simulink model "controller_ballcatcher_inv_kin_mind_timestamp"  (R2018b)
settings: Solver=FixedStepDiscrete  StartTime=0.0  StopTime=10.0  FixedStep=timing.T_optiTask  RelTol=1e-3
InitFcn:
  | iiwa_joint_trajectoryfollowingcontrol_rigid_parameters;
values from neighbouring files (symbols this model uses):
  estimator_init_struct = struct()    [init_estimator_struct.m]
  filter_tau_p_slow_T_1 = filter_tau_slow_T_1    [parameters.m]
  filter_tau_slow_T_1 = 1./(2*pi*[200;200;200;200;200;200;200])    [parameters.m]
  filter_theta_p_slow_T_1 = filter_tau_slow_T_1    [parameters.m]
  filter_theta_slow_T_1 = filter_tau_slow_T_1    [parameters.m]
  height_of_catch = 0.9    [init_estimator_struct.m]
  optitrack_data = struct()    [init_parabola.m]
  param_robot = struct()    [parameters.m]
  positions = struct()    [init_common_positions.m]
  sensor_torque_offset = [0.53;-0.095;-0.189;0.07;-0.058;0.0025;-0.12]    [parameters.m]
  timing = struct()    [parameters.m]
undefined symbols (not defined in the file or in its folder): param_controller
settings Model: TCT_ExtModeMexArgs=[128 131 86 77 1 1],16842832  SimulationMode=external  Creator=cha  LastModifiedBy=student
settings SolverCC: AutoInsertRateTranBlk=on
settings DataIOCC: LoggingToFile=on  LoggingFileName=benniii.mat
settings OptimizationCC: UseFloatMulNetSlope=on  PassReuseOutputArgsThreshold=0  LocalBlockOutputs=off  EfficientFloat2IntCast=on  OptimizeBlockOrder=speed  DifferentSizesBufferReuse=on
settings DebuggingCC: ParameterTunabilityLossMsg=error
settings HardwareCC: ProdLongLongMode=on
settings ModelReferenceCC: EnableParallelModelReferenceBuilds=on  ModelReferenceNumInstancesAllowed=Single
settings SFSimCC: SimUseLocalCustomCode=off  MATLABDynamicMemAlloc=off
settings RTWCC: SystemTargetFile=TwinCAT.tlc  GenCodeOnly=on  MakeCommand=make_tct  TemplateMakefile=tct_msbuild.tmf  Description=TwinCAT Target  GenerateReport=on  RTWUseLocalCustomCode=off  TargetLang=C++
settings RTWCC: CustomHeaderCode=|
  | #define fflush(stdout)
  | #define printf(...) m_spSrv->TcReportLog(ADSLOG_MSGTYPE_LOG,__VA_ARGS__)
settings CodeAppCC: ForceParamTrailComments=on  MaxIdLength=47  OperatorAnnotations=on  StateflowObjectComments=on  MATLABSourceComments=on
settings STFCustomTargetCC: TargetLangStandard=C++03 (ISO)  CompOptLevelCompliant=on  MATLABClassNameForMDSCustomization=Simulink.SoftwareTarget.TargetSpecificTriggerConfigurationBase  GRTInterface=on  SystemTargetFile=TwinCAT.tlc

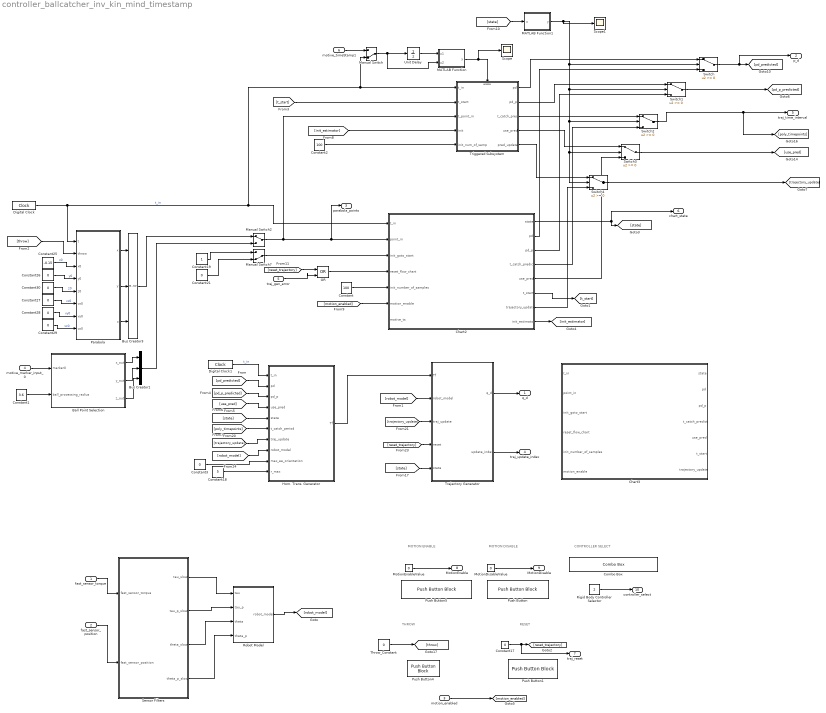
== system controller_ballcatcher_inv_kin_mind_timestamp ==
  note: THROW
  note: RESET
  note: MOTION ENABLE
  note: MOTION DISABLE
  note: CONTROLLER SELECT
  fast_sensor_torque : Inport
  fast_sensor_position : Inport  Port=2
  motion_enabled : Inport  Port=3
  motive_marker_input_0 : Inport  Port=4  OutDataTypeStr=Bus: Marker
  traj_gen_error : Inport  Port=5  OutDataTypeStr=boolean
  motive_timeStamp1 : Inport  Port=6
  Ball Point Selection : MATLAB Function  TreatAsAtomicUnit=on
  Bus Creator1 : BusCreator  Inputs=3
  Bus Creator3 : BusCreator  Inputs=3
  Chart2 : Stateflow chart  TreatAsAtomicUnit=on
  Chart3 : Subsystem
      mask help: Simulink:masks:GenSFuncDesc_MD
      mask Help: eval('feval(''rtwprivate'',''rtwhelpview'',''rtw_sfcn_block'')');
  Combo Box : ComboBox  WebBlockId=3098  SelectedLabel=2: Joint-based E/A Linearization
      settings: Values={{'1: Gravity Compensation q-based', '2: Joint-based E/A Linearization'}, [1 2]}
  Constant : Constant  Value=100
  Constant1 : Constant  Value=3.6
  Constant{3,17,21,26..30} (8 alike) : Constant  Value=0
  Constant18 : Constant  Value=5
  Constant19 : Constant
  Constant2 : Constant  Value=100
  Constant25 : Constant  Value=-0.15
  Digital Clock : DigitalClock  SampleTime=timing.T_optitrack
  Digital Clock1 : DigitalClock  SampleTime=timing.T_optiTask
  Hom. Trans. Generator : MATLAB Function  TreatAsAtomicUnit=on
  MATLAB Function : MATLAB Function  TreatAsAtomicUnit=on
  MATLAB Function1 : MATLAB Function  TreatAsAtomicUnit=on
  Manual Switch : ManualSwitch  CurrentSetting=0
  Manual Switch2 : ManualSwitch
  Manual Switch7 : ManualSwitch  CurrentSetting=0
  MotionDisableValue : Constant  Value=0
  MotionEnableValue : Constant  Value=0
  OR : Logic  Operator=OR  IconShape=distinctive  AllPortsSameDT=off  OutDataTypeStr=boolean
  Parabola : MATLAB Function  TreatAsAtomicUnit=on
  Push Button : PushButtonBlock  WebBlockId=3092  ButtonText=Motion disable
  Push Button1 : PushButtonBlock  WebBlockId=1355  ButtonText=Reset Trajectory
  Push Button4 : PushButtonBlock  WebBlockId=2019  ButtonText=Throw
  Push Button5 : PushButtonBlock  WebBlockId=3093  ButtonText=Motion enable
  Rigid Body Controller Selector : Constant  Value=2  OutDataTypeStr=uint32
  Robot Model : MATLAB Function  TreatAsAtomicUnit=on
  Scope : Scope
  Scope1 : Scope
  Sensor Filters : Subsystem
  Switch{,2..4} (4 alike) : Switch
  Switch1 : Switch  InputSameDT=on
  Throw_Constant : Constant  Value=0
  Trajectory Generator : MATLAB Function  TreatAsAtomicUnit=on
  Triggered Subsystem : Subsystem  TreatAsAtomicUnit=on
  Unit Delay : UnitDelay  SampleTime=-1
  q_d : Outport  PortDimensions=7  VectorParamsAs1DForOutWhenUnconnected=on
  p_d : Outport  Port=2  VectorParamsAs1DForOutWhenUnconnected=on
  parabola_points : Outport  Port=3  VectorParamsAs1DForOutWhenUnconnected=on
  traj_update_index : Outport  Port=4
  traj_time_interval : Outport  Port=5
  chart_state : Outport  Port=6
  traj_reset : Outport  Port=7
  MotionEnable : Outport  Port=8
  MotionDisable : Outport  Port=9
  controller_select : Outport  Port=10
  wires:
  motion_enabled/1 -> [motion_enabled]
  fast_sensor_torque/1 -> Sensor Filters/1(fast_sensor_torque)
  fast_sensor_position/1 -> Sensor Filters/2(fast_sensor_position)
  Sensor Filters/1(tau_slow) -> Robot Model/1(tau)
  Sensor Filters/2(tau_p_slow) -> Robot Model/2(tau_p)
  Sensor Filters/3(theta_slow) -> Robot Model/3(theta)
  Sensor Filters/4(theta_p_slow) -> Robot Model/4(theta_p)
  Robot Model/1(robot_model) -> [robot_model]
  [use_pred] -> Hom. Trans. Generator/4(use_pred)
  [pd_p_predicted] -> Hom. Trans. Generator/3(pd_p)
  [state] -> Hom. Trans. Generator/5(state)
  [pd_predicted] -> Hom. Trans. Generator/2(pd)
  Constant21/1 -> Manual Switch7/2
  Constant19/1 -> Manual Switch7/1
  motive_marker_input_0/1 -> Ball Point Selection/1(marker0)
  Hom. Trans. Generator/1(Tf) -> Trajectory Generator/1(Tf)
  Trajectory Generator/1(q_d) -> q_d/1
  Manual Switch7/1 -> Chart2/3(init_goto_start)
  Chart2/1(state) -> [state], chart_state/1
  Chart2/6(t_start) -> [t_start]
  Digital Clock/1 -> Manual Switch/2, Triggered Subsystem/1(t_in), Chart2/1(t_in), Parabola/1(t)  "t_in"
  Ball Point Selection/1(x_out) -> Bus Creator1/1
  Ball Point Selection/2(y_out) -> Bus Creator1/2
  Ball Point Selection/3(z_out) -> Bus Creator1/3
  [throw] -> Parabola/2(throw)
  Throw_Constant/1 -> [throw]
  Parabola/3(z) -> Bus Creator3/3
  Parabola/2(y) -> Bus Creator3/2
  Parabola/1(x) -> Bus Creator3/1
  Manual Switch2/1 -> Triggered Subsystem/3(t_point_in), Chart2/2(point_in), parabola_points/1
  Bus Creator3/1 -> Manual Switch2/1
  Bus Creator1/1 -> Manual Switch2/2
  Constant26/1 -> Parabola/4(y0)  "y0"
  Constant27/1 -> Parabola/6(vx0)  "vx0"
  Constant30/1 -> Parabola/5(z0)  "z0"
  Constant25/1 -> Parabola/3(x0)  "x0"
  Constant29/1 -> Parabola/8(vz0)  "vz0"
  Constant28/1 -> Parabola/7(vy0)  "vy0"
  [poly_timepoints] -> Hom. Trans. Generator/6(t_catch_period)
  [trajectory_update] -> Trajectory Generator/3(traj_update)
  [robot_model] -> Hom. Trans. Generator/8(robot_model)
  Constant/1 -> Chart2/5(init_number_of_samples)
  [trajectory_update] -> Hom. Trans. Generator/7(traj_update)
  Constant1/1 -> Ball Point Selection/2(ball_processing_radius)
  Constant3/1 -> Hom. Trans. Generator/9(max_ee_orientation)
  [reset_trajectory] -> Trajectory Generator/4(reset)
  [motion_enabled] -> Chart2/6(motion_enable)
  Constant18/1 -> Hom. Trans. Generator/10(r_max)
  [state] -> Trajectory Generator/5(state)
  Constant17/1 -> traj_reset/1, [reset_trajectory]
  OR/1 -> Chart2/4(reset_flow_chart)
  [reset_trajectory] -> OR/1
  traj_gen_error/1 -> OR/2
  Trajectory Generator/2(update_index) -> traj_update_index/1
  Digital Clock1/1 -> Hom. Trans. Generator/1(t_in)  "t_in"
  [robot_model] -> Trajectory Generator/2(robot_model)
  MotionDisableValue/1 -> MotionDisable/1
  MotionEnableValue/1 -> MotionEnable/1
  Rigid Body Controller Selector/1 -> controller_select/1
  [t_start] -> Triggered Subsystem/2(t_start)
  Chart2/8(init_estimator) -> [init_estimator]
  [init_estimator] -> Triggered Subsystem/4(init)
  Constant2/1 -> Triggered Subsystem/5(init_num_of_samp)
  Unit Delay/1 -> MATLAB Function/1(u1)
  Switch/1 -> p_d/1, [pd_predicted]
  Switch1/1 -> [pd_p_predicted]
  Switch2/1 -> [poly_timepoints], traj_time_interval/1
  Switch3/1 -> [use_pred]
  Triggered Subsystem/1(pd) -> Switch/1
  Triggered Subsystem/2(pd_p) -> Switch1/1
  Triggered Subsystem/4(use_pred) -> Switch3/1
  Triggered Subsystem/3(t_catch_pred) -> Switch2/1
  Triggered Subsystem/5(pred_update) -> Switch4/1
  Switch4/1 -> [trajectory_update]
  Chart2/2(pd) -> Switch/3
  Chart2/3(pd_p) -> Switch1/3
  Chart2/4(t_catch_predict) -> Switch2/3
  Chart2/5(use_pred) -> Switch3/3
  Chart2/7(trajectory_update) -> Switch4/3
  [state] -> MATLAB Function1/1(u)
  MATLAB Function1/1(y) -> Scope1/1, Switch4/2, Switch3/2, Switch2/2, Switch1/2, Switch/2
  MATLAB Function/1(y) -> Triggered Subsystem/Enable, Scope/1
  Manual Switch/1 -> Unit Delay/1, MATLAB Function/2(u2)
  motive_timeStamp1/1 -> Manual Switch/1

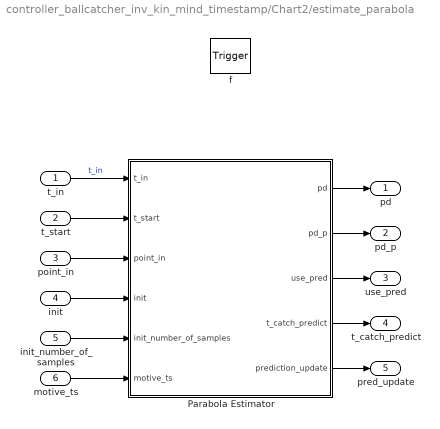
== system controller_ballcatcher_inv_kin_mind_timestamp/Chart2/estimate_parabola ==
  t_in : Inport  OutDataTypeStr=double  PortDimensions=1
  t_start : Inport  Port=2  OutDataTypeStr=double  PortDimensions=1
  point_in : Inport  Port=3  OutDataTypeStr=double  PortDimensions=3
  init : Inport  Port=4  OutDataTypeStr=double  PortDimensions=1
  init_number_of_samples : Inport  Port=5  OutDataTypeStr=double  PortDimensions=1
  motive_ts : Inport  Port=6  OutDataTypeStr=double  PortDimensions=1
  f : TriggerPort  TriggerType=function-call  VariantControl=(inherit)
      settings: CopyFcn=Stateflow.SLINSF.SimulinkMan.removeBlockPreDeleteFcn  PreDeleteFcn=Stateflow.SLINSF.SimulinkMan.unsafePredeleteFcn
  Parabola Estimator : MATLAB Function  TreatAsAtomicUnit=on
  pd : Outport  PortDimensions=3  VectorParamsAs1DForOutWhenUnconnected=on
  pd_p : Outport  Port=2  PortDimensions=3  VectorParamsAs1DForOutWhenUnconnected=on
  use_pred : Outport  Port=3  PortDimensions=1  VectorParamsAs1DForOutWhenUnconnected=on
  t_catch_predict : Outport  Port=4  PortDimensions=[1,2]  VectorParamsAs1DForOutWhenUnconnected=on
  pred_update : Outport  Port=5  VectorParamsAs1DForOutWhenUnconnected=on
  wires:
  init_number_of_samples/1 -> Parabola Estimator/5(init_number_of_samples)
  Parabola Estimator/5(prediction_update) -> pred_update/1
  init/1 -> Parabola Estimator/4(init)
  t_start/1 -> Parabola Estimator/2(t_start)
  point_in/1 -> Parabola Estimator/3(point_in)
  t_in/1 -> Parabola Estimator/1(t_in)  "t_in"
  Parabola Estimator/3(use_pred) -> use_pred/1
  Parabola Estimator/4(t_catch_predict) -> t_catch_predict/1
  Parabola Estimator/1(pd) -> pd/1
  Parabola Estimator/2(pd_p) -> pd_p/1
  motive_ts/1 -> Parabola Estimator/6(motive_ts)

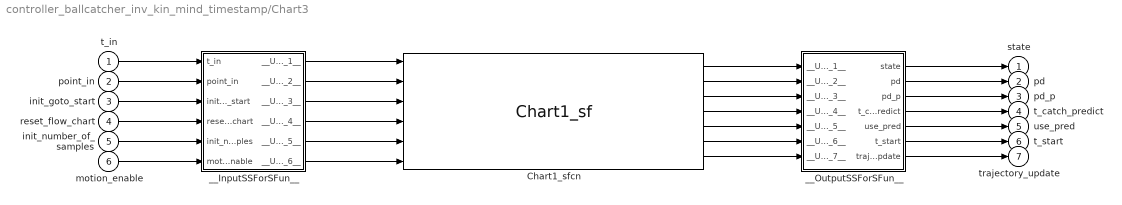
== system controller_ballcatcher_inv_kin_mind_timestamp/Chart3 ==
  t_in : Inport
  point_in : Inport  Port=2
  init_goto_start : Inport  Port=3
  reset_flow_chart : Inport  Port=4
  init_number_of_samples : Inport  Port=5
  motion_enable : Inport  Port=6
  Chart1_sfcn : S-Function  FunctionName=Chart1_sf  SFunctionModules=""  SFunctionDeploymentMode=off  EnableBusSupport=off  mask{rtw_sf_name=Chart1_sf, showVar=off}
      mask prompts: rtw_sf_name "Simulink:masks:GenSFuncName_MP"; showVar "Simulink:masks:GenSFuncShowModuleList_MP"
      mask help: Simulink:masks:GenSFuncDesc_MD
      mask init:
      | displist = '';
      | if ~strcmp(get_param(gcb, 'FunctionName'), rtw_sf_name);
      |   set_param(gcb, 'FunctionName', rtw_sf_name);
      | end
      | % Check if we are generating code
      | rtw_mode = false;
      | if strcmpi(get_param(bdroot(gcb),'SimulationStatus'),'Initializing')
      | 	rtw_mode = strcmpi(get_param(bdroot(gcb),'BuildingRTWCode'),'on') && ...
      | 		~strcmpi(get_param(bdroot(gcb),'TargetStyle'),'SimulationTarget');
      | end
      | if showVar || rtw_mode
      | 	if exist('rtwsfunc') == 2 | exist('rtwsfunc') == 6
      | 		tmplist = rtwsfunc(rtw_sf_name,gcb);
      | 		tmplist = DAStudio.message('Simulink:masks:GenSFuncListOfModules_IC', tmplist);
      | 	elseif showVar
      | 		tmplist1 = DAStudio.message('Simulink:masks:GenSFuncListOfModules_IC', '');
      |         tmplist2 = DAStudio.message('Simulink:masks:GenSFuncNotLicensed_IC');
      |         tmplist = [tmplist1 tmplist2];
      |  	end
      | end
      | if showVar
      |   displist = tmplist;
      | end
      settings: CopyFcn=|
      | if ~strcmp(get_param(gcb,'Linkstatus'),'none') && ...
      | ~strcmp(get_param(gcb,'Linkstatus'),'implicit')
      |   set_param(gcb,'LinkStatus','none');
      | end
      mask Help: eval('feval(''rtwprivate'',''rtwhelpview'',''rtw_sfcn_block'')');
      mask Display:
      | port_label('input',1,'t_in');
      | port_label('input',2,'point_in');
      | port_label('input',3,'init_goto_start');
      | port_label('input',4,'reset_flow_chart');
      | port_label('input',5,'init_number_of_samples');
      | port_label('input',6,'motion_enable');
      | port_label('output',1,'state');
      | port_label('output',2,'pd');
      | port_label('output',3,'pd_p');
      | port_label('output',4,'t_catch_predict');
      | port_label('output',5,'use_pred');
      | port_label('output',6,'t_start');
      | port_label('output',7,'trajectory_update');
  __InputSSForSFun__ : Subsystem
  __OutputSSForSFun__ : Subsystem
  state : Outport  VectorParamsAs1DForOutWhenUnconnected=on
  pd : Outport  Port=2  VectorParamsAs1DForOutWhenUnconnected=on
  pd_p : Outport  Port=3  VectorParamsAs1DForOutWhenUnconnected=on
  t_catch_predict : Outport  Port=4  VectorParamsAs1DForOutWhenUnconnected=on
  use_pred : Outport  Port=5  VectorParamsAs1DForOutWhenUnconnected=on
  t_start : Outport  Port=6  VectorParamsAs1DForOutWhenUnconnected=on
  trajectory_update : Outport  Port=7  VectorParamsAs1DForOutWhenUnconnected=on
  wires:
  __OutputSSForSFun__/7(trajectory_update) -> trajectory_update/1
  __OutputSSForSFun__/6(t_start) -> t_start/1
  __OutputSSForSFun__/5(use_pred) -> use_pred/1
  __OutputSSForSFun__/4(t_catch_predict) -> t_catch_predict/1
  __OutputSSForSFun__/3(pd_p) -> pd_p/1
  __OutputSSForSFun__/2(pd) -> pd/1
  __OutputSSForSFun__/1(state) -> state/1
  Chart1_sfcn/7 -> __OutputSSForSFun__/7(__UniqueInportName__7__)
  Chart1_sfcn/6 -> __OutputSSForSFun__/6(__UniqueInportName__6__)
  Chart1_sfcn/5 -> __OutputSSForSFun__/5(__UniqueInportName__5__)
  Chart1_sfcn/4 -> __OutputSSForSFun__/4(__UniqueInportName__4__)
  Chart1_sfcn/3 -> __OutputSSForSFun__/3(__UniqueInportName__3__)
  Chart1_sfcn/2 -> __OutputSSForSFun__/2(__UniqueInportName__2__)
  Chart1_sfcn/1 -> __OutputSSForSFun__/1(__UniqueInportName__1__)
  __InputSSForSFun__/6(__UniqueOutportName__6__) -> Chart1_sfcn/6
  __InputSSForSFun__/5(__UniqueOutportName__5__) -> Chart1_sfcn/5
  __InputSSForSFun__/4(__UniqueOutportName__4__) -> Chart1_sfcn/4
  __InputSSForSFun__/3(__UniqueOutportName__3__) -> Chart1_sfcn/3
  __InputSSForSFun__/2(__UniqueOutportName__2__) -> Chart1_sfcn/2
  __InputSSForSFun__/1(__UniqueOutportName__1__) -> Chart1_sfcn/1
  motion_enable/1 -> __InputSSForSFun__/6(motion_enable)
  init_number_of_samples/1 -> __InputSSForSFun__/5(init_number_of_samples)
  reset_flow_chart/1 -> __InputSSForSFun__/4(reset_flow_chart)
  init_goto_start/1 -> __InputSSForSFun__/3(init_goto_start)
  point_in/1 -> __InputSSForSFun__/2(point_in)
  t_in/1 -> __InputSSForSFun__/1(t_in)

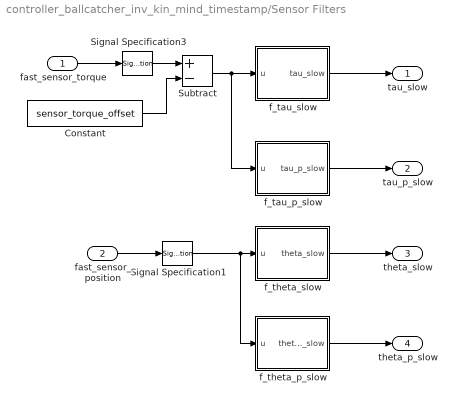
== system controller_ballcatcher_inv_kin_mind_timestamp/Sensor Filters ==
  fast_sensor_torque : Inport
  fast_sensor_position : Inport  Port=2
  Constant : Constant  Value=sensor_torque_offset
  Signal Specification1 : SignalSpecification  Dimensions=7
  Signal Specification3 : SignalSpecification  Dimensions=7
  Subtract : Sum  Inputs=+-
  f_tau_p_slow : MATLAB Function  TreatAsAtomicUnit=on
  f_tau_slow : MATLAB Function  TreatAsAtomicUnit=on
  f_theta_p_slow : MATLAB Function  TreatAsAtomicUnit=on
  f_theta_slow : MATLAB Function  TreatAsAtomicUnit=on
  tau_slow : Outport
  tau_p_slow : Outport  Port=2
  theta_slow : Outport  Port=3
  theta_p_slow : Outport  Port=4
  wires:
  fast_sensor_position/1 -> Signal Specification1/1
  Signal Specification1/1 -> f_theta_p_slow/1(u), f_theta_slow/1(u)
  f_theta_p_slow/1(theta_p_slow) -> theta_p_slow/1
  f_theta_slow/1(theta_slow) -> theta_slow/1
  f_tau_slow/1(tau_slow) -> tau_slow/1
  f_tau_p_slow/1(tau_p_slow) -> tau_p_slow/1
  Constant/1 -> Subtract/2
  Subtract/1 -> f_tau_p_slow/1(u), f_tau_slow/1(u)
  fast_sensor_torque/1 -> Signal Specification3/1
  Signal Specification3/1 -> Subtract/1

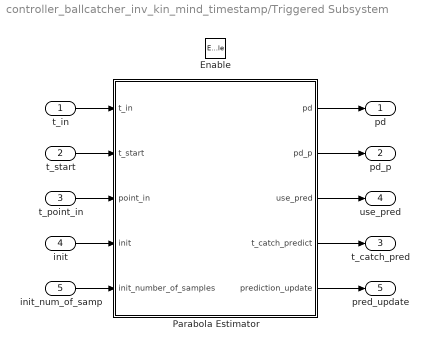
== system controller_ballcatcher_inv_kin_mind_timestamp/Triggered Subsystem ==
  t_in : Inport
  t_start : Inport  Port=2
  t_point_in : Inport  Port=3
  init : Inport  Port=4
  init_num_of_samp : Inport  Port=5
  Enable : EnablePort
  Parabola Estimator : MATLAB Function  TreatAsAtomicUnit=on
  pd : Outport
  pd_p : Outport  Port=2
  t_catch_pred : Outport  Port=3
  use_pred : Outport  Port=4
  pred_update : Outport  Port=5
  wires:
  t_in/1 -> Parabola Estimator/1(t_in)
  t_start/1 -> Parabola Estimator/2(t_start)
  t_point_in/1 -> Parabola Estimator/3(point_in)
  init/1 -> Parabola Estimator/4(init)
  init_num_of_samp/1 -> Parabola Estimator/5(init_number_of_samples)
  Parabola Estimator/1(pd) -> pd/1
  Parabola Estimator/5(prediction_update) -> pred_update/1
  Parabola Estimator/4(t_catch_predict) -> t_catch_pred/1
  Parabola Estimator/3(use_pred) -> use_pred/1
  Parabola Estimator/2(pd_p) -> pd_p/1

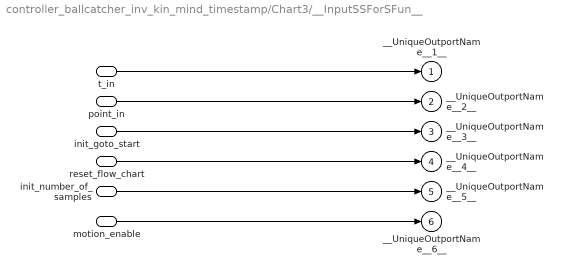
== system controller_ballcatcher_inv_kin_mind_timestamp/Chart3/__InputSSForSFun__ ==
  t_in : Inport
  point_in : Inport  Port=2
  init_goto_start : Inport  Port=3
  reset_flow_chart : Inport  Port=4
  init_number_of_samples : Inport  Port=5
  motion_enable : Inport  Port=6
  __UniqueOutportName__1__ : Outport
  __UniqueOutportName__2__ : Outport  Port=2
  __UniqueOutportName__3__ : Outport  Port=3
  __UniqueOutportName__4__ : Outport  Port=4
  __UniqueOutportName__5__ : Outport  Port=5
  __UniqueOutportName__6__ : Outport  Port=6
  wires:
  motion_enable/1 -> __UniqueOutportName__6__/1
  init_number_of_samples/1 -> __UniqueOutportName__5__/1
  reset_flow_chart/1 -> __UniqueOutportName__4__/1
  init_goto_start/1 -> __UniqueOutportName__3__/1
  point_in/1 -> __UniqueOutportName__2__/1
  t_in/1 -> __UniqueOutportName__1__/1

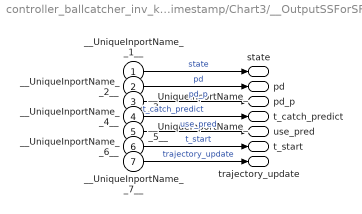
== system controller_ballcatcher_inv_kin_mind_timestamp/Chart3/__OutputSSForSFun__ ==
  __UniqueInportName__1__ : Inport
  __UniqueInportName__2__ : Inport  Port=2
  __UniqueInportName__3__ : Inport  Port=3
  __UniqueInportName__4__ : Inport  Port=4
  __UniqueInportName__5__ : Inport  Port=5
  __UniqueInportName__6__ : Inport  Port=6
  __UniqueInportName__7__ : Inport  Port=7
  state : Outport  VectorParamsAs1DForOutWhenUnconnected=on
  pd : Outport  Port=2  VectorParamsAs1DForOutWhenUnconnected=on
  pd_p : Outport  Port=3  VectorParamsAs1DForOutWhenUnconnected=on
  t_catch_predict : Outport  Port=4  VectorParamsAs1DForOutWhenUnconnected=on
  use_pred : Outport  Port=5  VectorParamsAs1DForOutWhenUnconnected=on
  t_start : Outport  Port=6  VectorParamsAs1DForOutWhenUnconnected=on
  trajectory_update : Outport  Port=7  VectorParamsAs1DForOutWhenUnconnected=on
  wires:
  __UniqueInportName__7__/1 -> trajectory_update/1  "trajectory_update"
  __UniqueInportName__6__/1 -> t_start/1  "t_start"
  __UniqueInportName__5__/1 -> use_pred/1  "use_pred"
  __UniqueInportName__4__/1 -> t_catch_predict/1  "t_catch_predict"
  __UniqueInportName__3__/1 -> pd_p/1  "pd_p"
  __UniqueInportName__2__/1 -> pd/1  "pd"
  __UniqueInportName__1__/1 -> state/1  "state"

== matlab function controller_ballcatcher_inv_kin_mind_timestamp/Parabola ==
  data: t input; x output; y output; z output; throw input; x0 input; y0 input; z0 input; vx0 input; vy0 input; vz0 input; optitrack_data parameter; param_controller parameter; timing parameter
function [x,y,z] = fcn(t,throw,x0,y0,z0,vx0,vy0,vz0,optitrack_data,param_controller,timing)
  
%   persistent t_throw_start throw_pers;
% 
%   if(isempty(t_throw_start))
%     t_throw_start=0;
%     throw_pers = 0;
%   end
%   
%   x = 0;
%   y = 0;
%   z = 0;
% 
%   if(throw)
%     t_throw_start = t+timing.T_optitrack;
%     throw_pers = 1;
%   end
%   
%   if(throw_pers && throw==0)
%     t_diff = t - t_throw_start;
% 
%     x = x0 + vx0*t_diff;
%     y = y0 + vy0*t_diff;
%     z = z0 + vz0*t_diff - (param_controller.g/2)*t_diff.^2;
%     
%     if z < (0.7)
%       throw_pers = 0;
%     end
%   end
  
  persistent t_throw_start throw_pers i;

  if(isempty(t_throw_start))
    t_throw_start=0;
    throw_pers = 0;
    i = 1;
  end
  
  x = 0;
  y = 0;
  z = 0;

  if(throw)
    t_throw_start = t+timing.T_optitrack;
    throw_pers = 1;
    i = 1;
  end
  
  if(throw_pers && throw==0)
    x = optitrack_data.x(i) + x0;
    y = optitrack_data.y(i) + y0;
    z = optitrack_data.z(i) + z0;
    
    i = i+1;
    
    if z < (0.7) && i > 100 % i > 100 to prevent stopping at the beginning if z is < 0.7
      throw_pers = 0;
    end
  end
end

== matlab function controller_ballcatcher_inv_kin_mind_timestamp/Ball Point Selection ==
  data: marker0 input; x_out output; y_out output; z_out output; ball_processing_radius input
function [x_out,y_out,z_out] = fcn(marker0,ball_processing_radius)
  x = marker0.x;
  y = marker0.y;
  z = marker0.z;
  
  r = sqrt(x^2+y^2);
  if(r > ball_processing_radius)
    x_out = 0;
    y_out = 0;
    z_out = 0;
  else
    x_out = x;
    y_out = y;
    z_out = z;
  end
end

== stateflow chart controller_ballcatcher_inv_kin_mind_timestamp/Chart2 ==
  state [pd,pd_p,use_pred,t_catch_predict,pred_update] = estimate_parabola(t_in,t_start,point_in,init,init_number_of_samples,motive_ts) [function] [commented out]
  state INIT
    entry:
    state=0;
    use_pred=0;
    trajectory_update = 0;
    t_catch_predict=[0,0];
    %pd=positions.candle;
    %pd_p=positions.candle_p;
  state INIT_GOTO_START
    entry:
    trajectory_update = 1;
    t_catch_predict=[t_in,t_in+0.5];
    pd=positions.start;
    pd_p=positions.start_p;
    during:
    trajectory_update = 0;
  state READY
    entry:
    state=1;
    trajectory_update = 0;
  state CATCH
    entry:
    t_catch_predict=[t_in+1,t_in+2];
    state=2;
    t_start=t_in;
    init_estimator=1;
    during:
    init_estimator=0;
  state GO_TO_START_FROM_NO_CATCH
    entry:
    trajectory_update = 1;
    state=4;
    t_catch_predict=[t_in,t_in+0.5];
    pd=positions.start;
    pd_p=positions.start_p;
    during:
    trajectory_update = 0;
  state NO_VALID_BALL_VALUE
    entry:
    state=3;
    use_pred=0;
    trajectory_update = 0;
  CATCH -> INIT [order 1] : [reset_flow_chart]
  (default) -> INIT
  NO_VALID_BALL_VALUE -> INIT [order 1] : [reset_flow_chart]
  INIT_GOTO_START -> INIT [order 1] : [reset_flow_chart]
  GO_TO_START_FROM_NO_CATCH -> INIT [order 1] : [reset_flow_chart]
  READY -> INIT [order 1] : [reset_flow_chart]
  INIT -> INIT_GOTO_START : [init_goto_start && motion_enable]
  INIT_GOTO_START -> READY [order 2] : [after(0.5,sec)]
  READY -> CATCH [order 2] : [isBallValueValid(point_in)]
  GO_TO_START_FROM_NO_CATCH -> READY [order 2] : [after(0.5,sec)]
  CATCH -> NO_VALID_BALL_VALUE [order 2] : [t_in > t_catch_predict(2)]
  NO_VALID_BALL_VALUE -> GO_TO_START_FROM_NO_CATCH [order 2] : [after(3,sec)]
  data: t_in function_input double size=1; t_start function_input double size=1; point_in function_input double size=1; init function_input double size=1; pd function_output double size=1; pd_p function_output double size=1; use_pred function_output double size=1; t_catch_predict function_output double size=1; pred_update function_output double size=1; init_number_of_samples function_input double size=1; motive_ts function_input double size=1; valid function_output size=1; data_point function_input size=3; state output; t_in input; point_in input; pd output; pd_p output; t_catch_predict output; use_pred output; positions parameter; t_start output; init_goto_start input; reset_flow_chart input; trajectory_update output; init_number_of_samples input; motion_enable input; motive_ts input; init_estimator output
  function valid  = isBallValueValid(data_point):
    | function valid  = isBallValueValid(data_point)
    | valid = ~(data_point(1) == 0 && data_point(2) == 0 && data_point(3) == 0);

== matlab function controller_ballcatcher_inv_kin_mind_timestamp/Chart2/estimate_parabola/Parabola Estimator ==
  data: t_in input; t_start input; point_in input; height_of_catch parameter; pd output; estimator_init_struct parameter; init input; pd_p output; use_pred output; t_catch_predict output; timing parameter; prediction_update output; init_number_of_samples input; motive_ts input
function [pd,pd_p,use_pred,t_catch_predict,prediction_update] = fcn(t_in,t_start,point_in,height_of_catch,estimator_init_struct,init,timing,init_number_of_samples,motive_ts)

    t_for_est = t_in-t_start;
    t_move_start = timing.T_optitrack*init_number_of_samples;
    t_start_g = t_start + t_move_start;
    prediction_update = 0;
    
    persistent use_pred_p t_catch_predict_p t_zd i pd__ pd_p__ t_in_last t_cnt blocked;
    if init || isempty(t_catch_predict_p)
        use_pred_p = 0;
        t_catch_predict_p = [t_start_g,t_start_g+1];
        t_zd = t_move_start+0.5;
        i = 0;
        pd__ = zeros(1,3);
        pd_p__ = zeros(1,3);
        t_in_last = t_in;
        t_cnt=0;
        blocked=false;
    end

    if i == 0
      if t_in >= t_catch_predict_p(1) && t_in <= t_catch_predict_p(2) && ~blocked
          blocked=true;
          use_pred_p = 1;
          g = 9.81; 

          [estimations,prediction_update]=estimate_parabola(t_for_est,point_in,estimator_init_struct,init);
          x0_est = estimations.x0_est;
          vx0_est = estimations.vx0_est;
          y0_est = estimations.y0_est;
          vy0_est = estimations.vy0_est;
          z0_est = estimations.z0_est;
          vz0_est = estimations.vz0_est;

          % parabola equations
          x = @(ti,x0_t,vx0_t) ( x0_t + vx0_t*ti );
          y = @(ti,y0_t,vy0_t) ( y0_t + vy0_t*ti );
          z = @(ti,z0_t,vz0_t) ( z0_t + vz0_t*ti - (g/2)*ti.^2 );

          % derivative equations
          x_p = @(vx0_t) ( vx0_t );
          y_p = @(vy0_t) ( vy0_t );
          z_p = @(ti,vz0_t) ( vz0_t - g*ti );

          % calculate time to catch
          za = -(g/2);
          zb = vz0_est;
          zc = z0_est;

          descriminant = -4*za*zc+4*za*height_of_catch+zb^2;
          if descriminant >= 0
             t_zd = -(zb+sqrt(descriminant))/(2*za);
          else
             %fprintf('WARNING: Complex solution for catching time');
          end

          % calculate catch coordinates
          x_out = x(t_zd,x0_est,vx0_est);
          y_out = y(t_zd,y0_est,vy0_est);
          z_out = z(t_zd,z0_est,vz0_est);
          pd__ = [x_out,y_out,z_out];

          % calculate derivatives (for ee orientation)
          x_out_p = x_p(vx0_est);
          y_out_p = y_p(vy0_est);
          z_out_p = z_p(t_zd,vz0_est);
          pd_p__ = [x_out_p,y_out_p,z_out_p]*(-1); % *(-1) because we want the
          % endeffector z-axis to point towards the ball

          t_catch_predict_p = [t_start_g,t_zd+t_start]; % -0.1 -> would be 100ms "time buffer"
      else
          use_pred_p = 0;
          [estimations,~]=estimate_parabola(t_for_est,point_in,estimator_init_struct,init);

          x_out = 0;
          y_out = 0;
          z_out = 0;
          pd__ = [x_out,y_out,z_out];

          x_out_p = 0;
          y_out_p = 0;
          z_out_p = 0;
          pd_p__ = [x_out_p,y_out_p,z_out_p]*(-1);
      end
    end
    
    % set outputs
    use_pred = use_pred_p;
    t_catch_predict = t_catch_predict_p;
    
    pd = pd__;
    pd_p = pd_p__;
    
    i = i+1;
   
    if i == timing.cycle_time_ratio
       i = 0;
    end
    
    if t_in == t_in_last
      t_cnt=t_cnt+1;
    else
      t_cnt=0;
    end
end

== matlab function controller_ballcatcher_inv_kin_mind_timestamp/MATLAB Function ==
  data: u1 input; y output; u2 input
function y = fcn(u1,u2)
  
  if u1==u2
    y=false;
  else
    y=true;
  end

== matlab function controller_ballcatcher_inv_kin_mind_timestamp/Triggered Subsystem/Parabola Estimator ==
  data: t_in input; t_start input; point_in input; height_of_catch parameter; pd output; estimator_init_struct parameter; init input; pd_p output; use_pred output; t_catch_predict output; timing parameter; prediction_update output; init_number_of_samples input
function [pd,pd_p,use_pred,t_catch_predict,prediction_update] = fcn(t_in,t_start,point_in,height_of_catch,estimator_init_struct,init,timing,init_number_of_samples)

    t_for_est = t_in-t_start;
    t_move_start = timing.T_optitrack*init_number_of_samples;
    t_start_g = t_start + t_move_start;
    prediction_update = 0;
    
    persistent use_pred_p t_catch_predict_p t_zd i pd__ pd_p__ t_in_last t_cnt blocked;
    if init || isempty(t_catch_predict_p)
        use_pred_p = 0;
        t_catch_predict_p = [t_start_g,t_start_g+1];
        t_zd = t_move_start+0.5;
        i = 0;
        pd__ = zeros(1,3);
        pd_p__ = zeros(1,3);
        t_in_last = t_in;
        t_cnt=0;
        blocked=false;
    end

    if i == 0
      if t_in >= t_catch_predict_p(1) && t_in <= t_catch_predict_p(2) && ~blocked
          blocked=true;
          use_pred_p = 1;
          g = 9.81; 

          [estimations,prediction_update]=estimate_parabola(t_for_est,point_in,estimator_init_struct,init);
          x0_est = estimations.x0_est;
          vx0_est = estimations.vx0_est;
          y0_est = estimations.y0_est;
          vy0_est = estimations.vy0_est;
          z0_est = estimations.z0_est;
          vz0_est = estimations.vz0_est;

          % parabola equations
          x = @(ti,x0_t,vx0_t) ( x0_t + vx0_t*ti );
          y = @(ti,y0_t,vy0_t) ( y0_t + vy0_t*ti );
          z = @(ti,z0_t,vz0_t) ( z0_t + vz0_t*ti - (g/2)*ti.^2 );

          % derivative equations
          x_p = @(vx0_t) ( vx0_t );
          y_p = @(vy0_t) ( vy0_t );
          z_p = @(ti,vz0_t) ( vz0_t - g*ti );

          % calculate time to catch
          za = -(g/2);
          zb = vz0_est;
          zc = z0_est;

          descriminant = -4*za*zc+4*za*height_of_catch+zb^2;
          if descriminant >= 0
             t_zd = -(zb+sqrt(descriminant))/(2*za);
          else
             %fprintf('WARNING: Complex solution for catching time');
          end

          % calculate catch coordinates
          x_out = x(t_zd,x0_est,vx0_est);
          y_out = y(t_zd,y0_est,vy0_est);
          z_out = z(t_zd,z0_est,vz0_est);
          pd__ = [x_out,y_out,z_out];

          % calculate derivatives (for ee orientation)
          x_out_p = x_p(vx0_est);
          y_out_p = y_p(vy0_est);
          z_out_p = z_p(t_zd,vz0_est);
          pd_p__ = [x_out_p,y_out_p,z_out_p]*(-1); % *(-1) because we want the
          % endeffector z-axis to point towards the ball

          t_catch_predict_p = [t_start_g,t_zd+t_start]; % -0.1 -> would be 100ms "time buffer"
      else
          use_pred_p = 0;
          [estimations,~]=estimate_parabola(t_for_est,point_in,estimator_init_struct,init);

          x_out = 0;
          y_out = 0;
          z_out = 0;
          pd__ = [x_out,y_out,z_out];

          x_out_p = 0;
          y_out_p = 0;
          z_out_p = 0;
          pd_p__ = [x_out_p,y_out_p,z_out_p]*(-1);
      end
    end
    
    % set outputs
    use_pred = use_pred_p;
    t_catch_predict = t_catch_predict_p;
    
    pd = pd__;
    pd_p = pd_p__;
    
    i = i+1;
   
    if i == timing.cycle_time_ratio
       i = 0;
    end
    
    if t_in == t_in_last
      t_cnt=t_cnt+1;
    else
      t_cnt=0;
    end
end

== matlab function controller_ballcatcher_inv_kin_mind_timestamp/Trajectory Generator ==
  data: Tf input; param_robot parameter; robot_model input; q_d output size=7; positions parameter; traj_update input; reset input; state input; update_index output
function [q_d,update_index]  = fcn(Tf,param_robot,robot_model,positions,traj_update,reset,state)
    persistent qf traj_update_index;
    
    n = 7;
    
    if isempty(qf)
      qf = robot_model.q;
      traj_update_index = 0;
    end
    
        
     if reset
       traj_update_index = 0;
       qf = robot_model.q;
     elseif traj_update
       traj_update_index = traj_update_index+1;

       if isequal(Tf,positions.T_candle)
          qf = zeros(n,1);
       else
          % if state==2 -> search for inv. kin. solution which is nearest
          % to current robot configuration
          [~,qf,~]=inverse_kinematics_analytic_schweng(Tf,param_robot,state==2,robot_model.q);
       end
     end
    
    q_d = qf;
    
    update_index = traj_update_index;

== matlab function controller_ballcatcher_inv_kin_mind_timestamp/Hom. Trans. Generator ==
  data: t_in input; pd input; pd_p input size=3; Tf output; use_pred input; state input; t_catch_period input; traj_update input; robot_model input; max_ee_orientation input; r_max input
function Tf   = trajectory_generator(t_in,pd,pd_p,use_pred,state,t_catch_period,traj_update,robot_model,max_ee_orientation,r_max)
    [Tf]=ball_follow_trajectory(pd,pd_p,use_pred,state,t_catch_period,t_in,traj_update,robot_model.H,max_ee_orientation,r_max);
end

== matlab function controller_ballcatcher_inv_kin_mind_timestamp/MATLAB Function1 ==
  data: u input; y output
function y = fcn(u)

y = u==2 || u==3;

== matlab function controller_ballcatcher_inv_kin_mind_timestamp/Sensor Filters/f_tau_slow ==
  data: u input; tau_slow output; param_controller parameter; filter_tau_slow_T_1 parameter
function tau_slow = func(u,param_controller, filter_tau_slow_T_1)
  persistent x;
  
  T_1=filter_tau_slow_T_1;
  alpha=exp(-param_controller.T_a./T_1);
  if(isempty(x))
    x=1./(1-alpha).*u;
    tau_slow=u;
  else
    tau_slow=(1-alpha).*x;
    x=alpha.*x+u;
  end
end

== matlab function controller_ballcatcher_inv_kin_mind_timestamp/Robot Model ==
  data: tau input; tau_p input; theta input; robot_model output Bus: robot_model; theta_p input; param_robot parameter; param_controller parameter
function robot_model = fcn(tau,tau_p,theta,theta_p,param_robot,param_controller)
  K=param_robot.K;
  
  robot_model=struct();
  %The calculation of q and q_p has to be performed with consistent cutoff
  %frequencies for the corresponding filters. The filters for q, q_p, tau
  %and tau_p have to have the same cutoff frequency.
  q=theta-diag(K).\tau;
  q_p=theta_p-diag(K).\tau_p;
  robot_model.q=q;
  robot_model.q_p=q_p;
  %Path Following Control with reverse kinematic
  robot_model.H=[iiwa_homogeneous_transformation_endeffector(q,param_robot);[0 0 0 1]];
  robot_model.J=iiwa_jacobian(q,param_robot);
  robot_model.J_p=iiwa_jacobian_p(q,q_p,param_robot);
  %If the singular perturbation controller is selected, the mass matrix has
  %to be modified according to Ott2008, Eq. (5.28).
  robot_model.M=iiwa_reduced_inertia_matrix(q,param_robot);
  %More efficient implementation for M+(I+K_tau)\B with diagonal
  %matrices K_tau and B: Only handle the diagonal elements.
  robot_model.M=robot_model.M+diag((1+param_controller.singular_perturbation.K_tau).\diag(param_robot.B));
  robot_model.C=iiwa_reduced_coriolis_matrix(q,q_p,param_robot);
  robot_model.g=iiwa_gravitational_force(q,param_robot);
end

== matlab function controller_ballcatcher_inv_kin_mind_timestamp/Sensor Filters/f_theta_slow ==
  data: u input; theta_slow output; param_controller parameter; filter_theta_slow_T_1 parameter
function theta_slow = func(u,param_controller, filter_theta_slow_T_1)
  persistent x;
  
  T_1=filter_theta_slow_T_1;
  alpha=exp(-param_controller.T_a./T_1);
  if(isempty(x))
    x=1./(1-alpha).*u;
    theta_slow=u;
  else
    theta_slow=(1-alpha).*x;
    x=alpha.*x+u;
  end
end

== matlab function controller_ballcatcher_inv_kin_mind_timestamp/Sensor Filters/f_tau_p_slow ==
  data: u input; tau_p_slow output; filter_tau_p_slow_T_1 parameter; param_controller parameter
function tau_p_slow = func(u,filter_tau_p_slow_T_1,param_controller)
  persistent x;
  
  T_1=filter_tau_p_slow_T_1;
  V=1/param_controller.T_a*(1-exp(-param_controller.T_a./T_1));
  if(isempty(x))
    x=-V.*u;
    tau_p_slow=zeros(size(u));
  else
    tau_p_slow=x+V.*u;
    x=exp(-param_controller.T_a./T_1).*x+(exp(-param_controller.T_a./T_1)-1).*V.*u;
  end
end

== matlab function controller_ballcatcher_inv_kin_mind_timestamp/Sensor Filters/f_theta_p_slow ==
  data: u input; theta_p_slow output; filter_theta_p_slow_T_1 parameter; param_controller parameter
function theta_p_slow = func(u,filter_theta_p_slow_T_1,param_controller)
  persistent x;
  
  T_1=filter_theta_p_slow_T_1;
  V=1/param_controller.T_a*(1-exp(-param_controller.T_a./T_1));
  if(isempty(x))
    x=-V.*u;
    theta_p_slow=zeros(size(u));
  else
    theta_p_slow=x+V.*u;
    x=exp(-param_controller.T_a./T_1).*x+(exp(-param_controller.T_a./T_1)-1).*V.*u;
  end
end
